simulink model "PhaseII_opalrt_NoProtection"  (Simulink 8.8)
settings: Solver=ode3  StartTime=0.0  StopTime=inf  FixedStep=Ts  RelTol=1e-5  EnableMultiTasking=on
PostLoadFcn:
  | %BESS ctrl
  | Kpf=0.005*3*12;
  | Kif=5*6;
  | 
  | Kpf1=0.005*3*12;
  | Kif1=5*6;
  | Kp_v=0.016*15*35;
  | Ki_v=12*25;
  | 
  | Kp_v1=0.016*15*35;
  | Ki_v1=12*25;
  | 
  | Vabc_B=12.47e3;
  | Vdc_ref=Vabc_B*2;
  | Kpwm=sqrt(2)*Vabc_B/Vdc_ref;
  | ZB=Vabc_B^2/1e6;
  | R=0.005*ZB;
  | Ibasefull=673/2*sqrt(2);
  | 
  | 
  | Ts_Control=1e-4;
  | ts=0.05;
  | delay=0.2;
  | offset=10e3;
  | t_plan=60;
  | t_monitor=.2;
  | t_mon=t_monitor;
  | scalingfactor=1;
  | x=0.5;
  | n=6;
  | %t_plan=1/15;
  | %t_monitor=10/900;
  | %t_mon=10/900;
  | 
  | %t_plan=1/5;
  | %t_monitor=10/300;
  | %t_mon=10/300;
  | %scalingfactor=1/300;
  | 
  | f0=60;
  | 
  | Pabc_B=1e6;
  | Iabc_B=Pabc_B*sqrt(2/3)/Vabc_B;  % pk value
  | Imax_1=2.5;
  | Ptrans_B=Pabc_B*200;
  | 
  | Vdc_ref=Vabc_B*2;
  | 
  | ZB=Vabc_B^2/Pabc_B;
  | L=0.1*ZB/2/pi/60;
  | R=0.1*ZB;
  | C=1/(4*pi^2*(2e3)^2*L);
  | 
  | LL=0.005*ZB/2/pi/60;
  | RR=0.005*ZB;
  | 
  | RC=0.02;
  | 
  | %%% Initial SOC %%%%
  | SOC_ini_BESS1=0.5;
  | ... (+223 lines)
InitFcn:
  | %BESS ctrl
  | Kpf=0.005*3*12;
  | Kif=5*6;
  | 
  | Kpf1=0.005*3*12;
  | Kif1=5*6;
  | Kp_v=0.016*15*35;
  | Ki_v=12*25;
  | 
  | Kp_v1=0.016*15*35;
  | Ki_v1=12*25;
  | 
  | Vabc_B=12.47e3;
  | Vdc_ref=Vabc_B*2;
  | Kpwm=sqrt(2)*Vabc_B/Vdc_ref;
  | ZB=Vabc_B^2/1e6;
  | R=0.005*ZB;
  | Ibasefull=673/2*sqrt(2);
  | 
  | 
  | Ts_Control=1e-4;
  | ts=0.05;
  | delay=0.2;
  | offset=10e3;
  | t_plan=60;
  | t_monitor=.2;
  | t_mon=t_monitor;
  | scalingfactor=1;
  | x=0.5;
  | n=6;
  | %t_plan=1/15;
  | %t_monitor=10/900;
  | %t_mon=10/900;
  | 
  | %t_plan=1/5;
  | %t_monitor=10/300;
  | %t_mon=10/300;
  | %scalingfactor=1/300;
  | 
  | f0=60;
  | 
  | Pabc_B=1e6;
  | Iabc_B=Pabc_B*sqrt(2/3)/Vabc_B;  % pk value
  | Imax_1=2.5;
  | Ptrans_B=Pabc_B*200;
  | 
  | Vdc_ref=Vabc_B*2;
  | 
  | ZB=Vabc_B^2/Pabc_B;
  | L=0.1*ZB/2/pi/60;
  | R=0.1*ZB;
  | C=1/(4*pi^2*(2e3)^2*L);
  | 
  | LL=0.005*ZB/2/pi/60;
  | RR=0.005*ZB;
  | 
  | RC=0.02;
  | 
  | %%% Initial SOC %%%%
  | SOC_ini_BESS1=0.5;
  | ... (+223 lines)
undefined symbols (not defined in the file): D1, Delta, DiscIntNeverNeededParam, Left, PG2ref, type, V
libraries: powerlib x220, powerlib_meascontrol x82, dspstat3 x54, dsparch4 x43, dspswit3 x24, simulink x19, simulink_extras x12, powerlib_extras x11, ssn_lib x7, artemis x6, rtlab x5, rtio_generic_dnp3 x5
(part 7 of 9)

== system PhaseII_opalrt_NoProtection/SM_System/Subsystem3/Fault ==
  In7 : Inport
  Breaker : powerlib/Elements/Breaker  InitialState=0  SwitchingTimes="[1/60  5/60]"  External=on  BreakerResistance=0.001  SnubberResistance=1e6  SnubberCapacitance=inf  Measurements=None  MoreParameters=on  NoBreakLoop=off
  Breaker1 : powerlib/Elements/Breaker  InitialState=0  SwitchingTimes="[1/60  5/60]"  External=on  BreakerResistance=0.001  SnubberResistance=1e6  SnubberCapacitance=inf  Measurements=None  MoreParameters=on  NoBreakLoop=off
  Breaker2 : powerlib/Elements/Breaker  InitialState=0  SwitchingTimes="[1/60  5/60]"  External=on  BreakerResistance=0.001  SnubberResistance=1e6  SnubberCapacitance=inf  Measurements=None  MoreParameters=on  NoBreakLoop=off
  In1 : PMIOPort  Port=1  Side=Left
  In2 : PMIOPort  Port=2  Side=Right
  In3 : PMIOPort  Port=3  Side=Left
  In4 : PMIOPort  Port=4  Side=Right
  In5 : PMIOPort  Port=5  Side=Left
  In6 : PMIOPort  Port=6  Side=Right
  wires:
  In7/1 -> Breaker1/1, Breaker2/1, Breaker/1
  connections:
  Breaker2/LConn1 -- In5/RConn1
  Breaker2/RConn1 -- In6/RConn1
  Breaker1/RConn1 -- In4/RConn1
  Breaker1/LConn1 -- In3/RConn1
  Breaker/RConn1 -- In2/RConn1
  Breaker/LConn1 -- In1/RConn1

== system PhaseII_opalrt_NoProtection/SM_System/Subsystem4/Fault ==
  In7 : Inport
  Breaker : powerlib/Elements/Breaker  InitialState=0  SwitchingTimes="[1/60  5/60]"  External=on  BreakerResistance=0.001  SnubberResistance=1e6  SnubberCapacitance=inf  Measurements=None  MoreParameters=on  NoBreakLoop=off
  Breaker1 : powerlib/Elements/Breaker  InitialState=0  SwitchingTimes="[1/60  5/60]"  External=on  BreakerResistance=0.001  SnubberResistance=1e6  SnubberCapacitance=inf  Measurements=None  MoreParameters=on  NoBreakLoop=off
  Breaker2 : powerlib/Elements/Breaker  InitialState=0  SwitchingTimes="[1/60  5/60]"  External=on  BreakerResistance=0.001  SnubberResistance=1e6  SnubberCapacitance=inf  Measurements=None  MoreParameters=on  NoBreakLoop=off
  In1 : PMIOPort  Port=1  Side=Left
  In2 : PMIOPort  Port=2  Side=Right
  In3 : PMIOPort  Port=3  Side=Left
  In4 : PMIOPort  Port=4  Side=Right
  In5 : PMIOPort  Port=5  Side=Left
  In6 : PMIOPort  Port=6  Side=Right
  wires:
  In7/1 -> Breaker/1, Breaker2/1, Breaker1/1
  connections:
  Breaker/LConn1 -- In1/RConn1
  Breaker/RConn1 -- In2/RConn1
  Breaker1/LConn1 -- In3/RConn1
  Breaker1/RConn1 -- In4/RConn1
  Breaker2/RConn1 -- In6/RConn1
  Breaker2/LConn1 -- In5/RConn1

== system PhaseII_opalrt_NoProtection/SS_LocalControl/BESS1/PI_Vd1 ==
  Error : Inport
  T_islanding : Inport  Port=2
  Add : Sum
  Add1 : Sum  Inputs=+-
  Constant25 : Constant  Value=4
  D2 : Scope  NumInputPorts=2
  Delay : Delay  DelayLength=1
  Embedded MATLAB Function1 : MATLAB Function  TreatAsAtomicUnit=on
  Integrator : Integrator  ExternalReset=rising  InitialConditionSource=external  LimitOutput=on  UpperSaturationLimit=Iabc_B*BESS_limit  LowerSaturationLimit=-Iabc_B*BESS_limit
  K : Gain
  K1 : Gain
  K2 : Gain  Gain=Vabc_B
  K3 : Gain  Gain=-1
  Ki1 : Gain  Gain=Kif/1.2
  Kp1 : Gain  Gain=Kpf/1.2
  Logical Operator : Logic  AllPortsSameDT=off  OutDataTypeStr=boolean
  PLL : powerlib_meascontrol/PLL/PLL  Fmin=58  Par_Init=[0, 60]  ParK=[180, 3200, 1]  TcD=1e-4  MaxRateChangeFreq=12  FilterCutOffFreq=25  Ts=0  AGC=on
  Relational Operator : RelationalOperator  Operator=<  OutDataTypeStr=boolean  ZeroCross=off  RndMeth=Nearest
  Relational Operator1 : RelationalOperator  Operator=>  OutDataTypeStr=boolean  ZeroCross=off  RndMeth=Nearest
  Out : Outport
  wires:
  K1/1 -> Relational Operator1/1, Relational Operator/1, Out/1
  Logical Operator/1 -> D2/1, Embedded MATLAB Function1/2(enable)
  Relational Operator/1 -> Logical Operator/1
  Relational Operator1/1 -> Logical Operator/2
  K3/1 -> Relational Operator1/2
  Embedded MATLAB Function1/1(dout) -> Integrator/1
  Add/1 -> K1/1
  K/1 -> Kp1/1, Ki1/1
  Ki1/1 -> Embedded MATLAB Function1/1(din)
  Kp1/1 -> Add1/2, Add/1
  Integrator/1 -> Add/2
  Constant25/1 -> K3/1, Relational Operator/2
  Error/1 -> D2/2, K/1
  T_islanding/1 -> Integrator/2
  Delay/1 -> Integrator/3
  [Ddg] -> Add1/1
  Add1/1 -> Delay/1

== system PhaseII_opalrt_NoProtection/SS_LocalControl/BESS1/PI_Vd10 ==
  Error : Inport
  T_islanding : Inport  Port=2
  Add : Sum
  Add1 : Sum  Inputs=+-
  Constant25 : Constant  Value=6
  D2 : Scope  NumInputPorts=2
  Delay : Delay  DelayLength=1
  Embedded MATLAB Function1 : MATLAB Function  TreatAsAtomicUnit=on
  Integrator1 : Integrator  ExternalReset=rising  InitialConditionSource=external  LimitOutput=on  UpperSaturationLimit=1  LowerSaturationLimit=-1
  K : Gain
  K1 : Gain
  K2 : Gain  Gain=Vabc_B
  K3 : Gain  Gain=-1
  Ki1 : Gain  Gain=Ki_v
  Kp1 : Gain  Gain=Kp_v
  Logical Operator : Logic  AllPortsSameDT=off  OutDataTypeStr=boolean
  PLL : powerlib_meascontrol/PLL/PLL  Fmin=58  Par_Init=[0, 60]  ParK=[180, 3200, 1]  TcD=1e-4  MaxRateChangeFreq=12  FilterCutOffFreq=25  Ts=0  AGC=on
  Relational Operator : RelationalOperator  Operator=<  OutDataTypeStr=boolean  ZeroCross=off  RndMeth=Nearest
  Relational Operator1 : RelationalOperator  Operator=>  OutDataTypeStr=boolean  ZeroCross=off  RndMeth=Nearest
  Out : Outport
  wires:
  Error/1 -> K/1, D2/2
  Constant25/1 -> Relational Operator/2, K3/1
  Integrator1/1 -> D2/1, Add/2
  Kp1/1 -> Add1/2, Add/1
  Ki1/1 -> Embedded MATLAB Function1/1(din)
  K/1 -> Ki1/1, Kp1/1
  Add/1 -> K1/1
  K3/1 -> Relational Operator1/2
  Relational Operator1/1 -> Logical Operator/2
  Relational Operator/1 -> Logical Operator/1
  Logical Operator/1 -> Embedded MATLAB Function1/2(enable)
  K1/1 -> Out/1, Relational Operator/1, Relational Operator1/1
  Embedded MATLAB Function1/1(dout) -> Integrator1/1
  T_islanding/1 -> Integrator1/2
  [Iq_ref_ini] -> Add1/1
  Add1/1 -> Delay/1
  Delay/1 -> Integrator1/3

== system PhaseII_opalrt_NoProtection/SS_LocalControl/BESS1/PI_Vd11 ==
  Error : Inport
  T_islanding : Inport  Port=2
  Add : Sum
  Add1 : Sum  Inputs=+-
  Constant25 : Constant  Value=4
  D2 : Scope  NumInputPorts=2
  Delay : Delay  DelayLength=1
  Embedded MATLAB Function1 : MATLAB Function  TreatAsAtomicUnit=on
  Integrator : Integrator  ExternalReset=rising  InitialConditionSource=external  LimitOutput=on  UpperSaturationLimit=Iabc_B*BESS_limit  LowerSaturationLimit=-Iabc_B*BESS_limit
  K : Gain
  K1 : Gain
  K2 : Gain  Gain=Vabc_B
  K3 : Gain  Gain=-1
  Ki1 : Gain  Gain=Kif/1.2
  Kp1 : Gain  Gain=Kpf/1.2
  Logical Operator : Logic  AllPortsSameDT=off  OutDataTypeStr=boolean
  PLL : powerlib_meascontrol/PLL/PLL  Fmin=58  Par_Init=[0, 60]  ParK=[180, 3200, 1]  TcD=1e-4  MaxRateChangeFreq=12  FilterCutOffFreq=25  Ts=0  AGC=on
  Relational Operator : RelationalOperator  Operator=<  OutDataTypeStr=boolean  ZeroCross=off  RndMeth=Nearest
  Relational Operator1 : RelationalOperator  Operator=>  OutDataTypeStr=boolean  ZeroCross=off  RndMeth=Nearest
  Out : Outport
  wires:
  K1/1 -> Relational Operator1/1, Relational Operator/1, Out/1
  Logical Operator/1 -> D2/1, Embedded MATLAB Function1/2(enable)
  Relational Operator/1 -> Logical Operator/1
  Relational Operator1/1 -> Logical Operator/2
  K3/1 -> Relational Operator1/2
  Embedded MATLAB Function1/1(dout) -> Integrator/1
  Add/1 -> K1/1
  K/1 -> Kp1/1, Ki1/1
  Ki1/1 -> Embedded MATLAB Function1/1(din)
  Kp1/1 -> Add1/2, Add/1
  Integrator/1 -> Add/2
  Constant25/1 -> K3/1, Relational Operator/2
  Error/1 -> D2/2, K/1
  T_islanding/1 -> Integrator/2
  Delay/1 -> Integrator/3
  [Dqg] -> Add1/1
  Add1/1 -> Delay/1

== system PhaseII_opalrt_NoProtection/SS_LocalControl/BESS1/PI_Vd2 ==
  Error : Inport
  Add : Sum
  Constant25 : Constant
  D2 : Scope  NumInputPorts=2
  Embedded MATLAB Function1 : MATLAB Function  TreatAsAtomicUnit=on
  Integrator : Integrator  ZeroCross=off
  K : Gain
  K1 : Gain
  K2 : Gain  Gain=Vabc_B
  K3 : Gain  Gain=-1
  Ki1 : Gain  Gain=Kif/1.2/1000
  Kp1 : Gain  Gain=Kpf/1.2
  Logical Operator : Logic  AllPortsSameDT=off  OutDataTypeStr=boolean
  PLL : powerlib_meascontrol/PLL/PLL  Fmin=58  Par_Init=[0, 60]  ParK=[180, 3200, 1]  TcD=1e-4  MaxRateChangeFreq=12  FilterCutOffFreq=25  Ts=0  AGC=on
  Relational Operator : RelationalOperator  Operator=<  OutDataTypeStr=boolean  ZeroCross=off  RndMeth=Nearest
  Relational Operator1 : RelationalOperator  Operator=>  OutDataTypeStr=boolean  ZeroCross=off  RndMeth=Nearest
  Out : Outport
  wires:
  K1/1 -> Relational Operator1/1, Relational Operator/1, Out/1
  Logical Operator/1 -> D2/1, Embedded MATLAB Function1/2(enable)
  Relational Operator/1 -> Logical Operator/1
  Relational Operator1/1 -> Logical Operator/2
  K3/1 -> Relational Operator1/2
  Embedded MATLAB Function1/1(dout) -> Integrator/1
  Add/1 -> K1/1
  K/1 -> Kp1/1, Ki1/1
  Ki1/1 -> Embedded MATLAB Function1/1(din)
  Kp1/1 -> Add/1
  Integrator/1 -> Add/2
  Constant25/1 -> K3/1, Relational Operator/2
  Error/1 -> D2/2, K/1

== system PhaseII_opalrt_NoProtection/SS_LocalControl/BESS1/PI_Vd3 ==
  Error : Inport
  Add : Sum
  Constant25 : Constant
  D2 : Scope  NumInputPorts=2
  Embedded MATLAB Function1 : MATLAB Function  TreatAsAtomicUnit=on
  Integrator : Integrator  ZeroCross=off
  K : Gain
  K1 : Gain
  K2 : Gain  Gain=Vabc_B
  K3 : Gain  Gain=-1
  Ki1 : Gain  Gain=Kif/1.2/1000
  Kp1 : Gain  Gain=Kpf/1.2
  Logical Operator : Logic  AllPortsSameDT=off  OutDataTypeStr=boolean
  PLL : powerlib_meascontrol/PLL/PLL  Fmin=58  Par_Init=[0, 60]  ParK=[180, 3200, 1]  TcD=1e-4  MaxRateChangeFreq=12  FilterCutOffFreq=25  Ts=0  AGC=on
  Relational Operator : RelationalOperator  Operator=<  OutDataTypeStr=boolean  ZeroCross=off  RndMeth=Nearest
  Relational Operator1 : RelationalOperator  Operator=>  OutDataTypeStr=boolean  ZeroCross=off  RndMeth=Nearest
  Out : Outport
  wires:
  K1/1 -> Relational Operator1/1, Relational Operator/1, Out/1
  Logical Operator/1 -> D2/1, Embedded MATLAB Function1/2(enable)
  Relational Operator/1 -> Logical Operator/1
  Relational Operator1/1 -> Logical Operator/2
  K3/1 -> Relational Operator1/2
  Embedded MATLAB Function1/1(dout) -> Integrator/1
  Add/1 -> K1/1
  K/1 -> Kp1/1, Ki1/1
  Ki1/1 -> Embedded MATLAB Function1/1(din)
  Kp1/1 -> Add/1
  Integrator/1 -> Add/2
  Constant25/1 -> K3/1, Relational Operator/2
  Error/1 -> D2/2, K/1

== system PhaseII_opalrt_NoProtection/SS_LocalControl/BESS1/PI_Vd5 ==
  Error : Inport
  Add : Sum
  Constant25 : Constant  Value=2
  D2 : Scope  NumInputPorts=2
  Embedded MATLAB Function1 : MATLAB Function  TreatAsAtomicUnit=on
  Integrator : Integrator  ZeroCross=off
  K : Gain
  K1 : Gain
  K2 : Gain  Gain=Vabc_B
  K3 : Gain  Gain=-1
  Ki1 : Gain  Gain=Ki_v
  Kp1 : Gain  Gain=Kp_v
  Logical Operator : Logic  AllPortsSameDT=off  OutDataTypeStr=boolean
  PLL : powerlib_meascontrol/PLL/PLL  Fmin=58  Par_Init=[0, 60]  ParK=[180, 3200, 1]  TcD=1e-4  MaxRateChangeFreq=12  FilterCutOffFreq=25  Ts=0  AGC=on
  Relational Operator : RelationalOperator  Operator=<  OutDataTypeStr=boolean  ZeroCross=off  RndMeth=Nearest
  Relational Operator1 : RelationalOperator  Operator=>  OutDataTypeStr=boolean  ZeroCross=off  RndMeth=Nearest
  Out : Outport
  wires:
  Error/1 -> K/1, D2/2
  Constant25/1 -> Relational Operator/2, K3/1
  Integrator/1 -> Add/2
  Kp1/1 -> Add/1
  Ki1/1 -> Embedded MATLAB Function1/1(din)
  K/1 -> Ki1/1, Kp1/1
  Add/1 -> K1/1
  Embedded MATLAB Function1/1(dout) -> Integrator/1
  K3/1 -> Relational Operator1/2
  Relational Operator1/1 -> Logical Operator/2
  Relational Operator/1 -> Logical Operator/1
  Logical Operator/1 -> Embedded MATLAB Function1/2(enable), D2/1
  K1/1 -> Out/1, Relational Operator/1, Relational Operator1/1

== system PhaseII_opalrt_NoProtection/SS_LocalControl/BESS1/PI_Vd6 ==
  Error : Inport
  Add : Sum
  Constant25 : Constant  Value=2
  D2 : Scope  NumInputPorts=2
  Embedded MATLAB Function1 : MATLAB Function  TreatAsAtomicUnit=on
  Integrator : Integrator  ZeroCross=off
  K : Gain
  K1 : Gain
  K2 : Gain  Gain=Vabc_B
  K3 : Gain  Gain=-1
  Ki1 : Gain  Gain=Ki_v
  Kp1 : Gain  Gain=Kp_v
  Logical Operator : Logic  AllPortsSameDT=off  OutDataTypeStr=boolean
  PLL : powerlib_meascontrol/PLL/PLL  Fmin=58  Par_Init=[0, 60]  ParK=[180, 3200, 1]  TcD=1e-4  MaxRateChangeFreq=12  FilterCutOffFreq=25  Ts=0  AGC=on
  Relational Operator : RelationalOperator  Operator=<  OutDataTypeStr=boolean  ZeroCross=off  RndMeth=Nearest
  Relational Operator1 : RelationalOperator  Operator=>  OutDataTypeStr=boolean  ZeroCross=off  RndMeth=Nearest
  Out : Outport
  wires:
  Error/1 -> K/1, D2/2
  Constant25/1 -> Relational Operator/2, K3/1
  Integrator/1 -> Add/2
  Kp1/1 -> Add/1
  Ki1/1 -> Embedded MATLAB Function1/1(din)
  K/1 -> Ki1/1, Kp1/1
  Add/1 -> K1/1
  Embedded MATLAB Function1/1(dout) -> Integrator/1
  K3/1 -> Relational Operator1/2
  Relational Operator1/1 -> Logical Operator/2
  Relational Operator/1 -> Logical Operator/1
  Logical Operator/1 -> Embedded MATLAB Function1/2(enable), D2/1
  K1/1 -> Out/1, Relational Operator/1, Relational Operator1/1

== system PhaseII_opalrt_NoProtection/SS_LocalControl/BESS1/PI_Vd7 ==
  Error : Inport
  T_islanding : Inport  Port=2
  Add : Sum
  Add1 : Sum  Inputs=+-
  Constant25 : Constant
  D2 : Scope  NumInputPorts=2
  Delay : Delay  DelayLength=1
  Embedded MATLAB Function1 : MATLAB Function  TreatAsAtomicUnit=on
  Integrator : Integrator  ExternalReset=falling  InitialConditionSource=external  LimitOutput=on  UpperSaturationLimit=Iabc_B*BESS_limit  LowerSaturationLimit=-Iabc_B*BESS_limit
  K : Gain
  K1 : Gain
  K2 : Gain  Gain=Vabc_B
  K3 : Gain  Gain=-1
  Ki1 : Gain  Gain=Kif
  Kp1 : Gain  Gain=Kpf
  Logical Operator : Logic  AllPortsSameDT=off  OutDataTypeStr=boolean
  PLL : powerlib_meascontrol/PLL/PLL  Fmin=58  Par_Init=[0, 60]  ParK=[180, 3200, 1]  TcD=1e-4  MaxRateChangeFreq=12  FilterCutOffFreq=25  Ts=0  AGC=on
  Relational Operator : RelationalOperator  Operator=<  OutDataTypeStr=boolean  ZeroCross=off  RndMeth=Nearest
  Relational Operator1 : RelationalOperator  Operator=>  OutDataTypeStr=boolean  ZeroCross=off  RndMeth=Nearest
  Out : Outport
  wires:
  K1/1 -> Relational Operator1/1, Relational Operator/1, Out/1
  Logical Operator/1 -> D2/1, Embedded MATLAB Function1/2(enable)
  Relational Operator/1 -> Logical Operator/1
  Relational Operator1/1 -> Logical Operator/2
  K3/1 -> Relational Operator1/2
  Embedded MATLAB Function1/1(dout) -> Integrator/1
  Add/1 -> K1/1
  K/1 -> Kp1/1, Ki1/1
  Ki1/1 -> Embedded MATLAB Function1/1(din)
  Kp1/1 -> Add1/2, Add/1
  Integrator/1 -> Add/2
  Constant25/1 -> K3/1, Relational Operator/2
  Error/1 -> D2/2, K/1
  T_islanding/1 -> Integrator/2
  Delay/1 -> Integrator/3
  [Ddi] -> Add1/1
  Add1/1 -> Delay/1

== system PhaseII_opalrt_NoProtection/SS_LocalControl/BESS1/PI_Vd8 ==
  Error : Inport
  T_islanding : Inport  Port=2
  Add : Sum
  Add1 : Sum  Inputs=+-
  Constant25 : Constant  Value=4
  D2 : Scope  NumInputPorts=2
  Delay : Delay  DelayLength=1
  Embedded MATLAB Function1 : MATLAB Function  TreatAsAtomicUnit=on
  Integrator1 : Integrator  ExternalReset=rising  InitialConditionSource=external  LimitOutput=on  UpperSaturationLimit=2.2  LowerSaturationLimit=-2.2
  K : Gain
  K1 : Gain
  K2 : Gain  Gain=Vabc_B
  K3 : Gain  Gain=-1
  Ki1 : Gain  Gain=Ki_v
  Kp1 : Gain  Gain=Kp_v
  Logical Operator : Logic  AllPortsSameDT=off  OutDataTypeStr=boolean
  PLL : powerlib_meascontrol/PLL/PLL  Fmin=58  Par_Init=[0, 60]  ParK=[180, 3200, 1]  TcD=1e-4  MaxRateChangeFreq=12  FilterCutOffFreq=25  Ts=0  AGC=on
  Relational Operator : RelationalOperator  Operator=<  OutDataTypeStr=boolean  ZeroCross=off  RndMeth=Nearest
  Relational Operator1 : RelationalOperator  Operator=>  OutDataTypeStr=boolean  ZeroCross=off  RndMeth=Nearest
  Out : Outport
  wires:
  Error/1 -> K/1, D2/2
  Constant25/1 -> Relational Operator/2, K3/1
  Integrator1/1 -> D2/1, Add/2
  Kp1/1 -> Add1/2, Add/1
  Ki1/1 -> Embedded MATLAB Function1/1(din)
  K/1 -> Ki1/1, Kp1/1
  Add/1 -> K1/1
  K3/1 -> Relational Operator1/2
  Relational Operator1/1 -> Logical Operator/2
  Relational Operator/1 -> Logical Operator/1
  Logical Operator/1 -> Embedded MATLAB Function1/2(enable)
  K1/1 -> Out/1, Relational Operator/1, Relational Operator1/1
  Embedded MATLAB Function1/1(dout) -> Integrator1/1
  T_islanding/1 -> Integrator1/2
  [Id_ref_ini] -> Add1/1
  Add1/1 -> Delay/1
  Delay/1 -> Integrator1/3

== system PhaseII_opalrt_NoProtection/SS_LocalControl/BESS1/PI_Vd9 ==
  Error : Inport
  T_islanding : Inport  Port=2
  Add : Sum
  Add1 : Sum  Inputs=+-
  Constant25 : Constant
  D2 : Scope  NumInputPorts=2
  Delay : Delay  DelayLength=1
  Embedded MATLAB Function1 : MATLAB Function  TreatAsAtomicUnit=on
  Integrator : Integrator  ExternalReset=falling  InitialConditionSource=external  LimitOutput=on  UpperSaturationLimit=Iabc_B*BESS_limit  LowerSaturationLimit=-Iabc_B*BESS_limit
  K : Gain
  K1 : Gain
  K2 : Gain  Gain=Vabc_B
  K3 : Gain  Gain=-1
  Ki1 : Gain  Gain=Kif
  Kp1 : Gain  Gain=Kpf
  Logical Operator : Logic  AllPortsSameDT=off  OutDataTypeStr=boolean
  PLL : powerlib_meascontrol/PLL/PLL  Fmin=58  Par_Init=[0, 60]  ParK=[180, 3200, 1]  TcD=1e-4  MaxRateChangeFreq=12  FilterCutOffFreq=25  Ts=0  AGC=on
  Relational Operator : RelationalOperator  Operator=<  OutDataTypeStr=boolean  ZeroCross=off  RndMeth=Nearest
  Relational Operator1 : RelationalOperator  Operator=>  OutDataTypeStr=boolean  ZeroCross=off  RndMeth=Nearest
  Out : Outport
  wires:
  K1/1 -> Relational Operator1/1, Relational Operator/1, Out/1
  Logical Operator/1 -> D2/1, Embedded MATLAB Function1/2(enable)
  Relational Operator/1 -> Logical Operator/1
  Relational Operator1/1 -> Logical Operator/2
  K3/1 -> Relational Operator1/2
  Embedded MATLAB Function1/1(dout) -> Integrator/1
  Add/1 -> K1/1
  K/1 -> Kp1/1, Ki1/1
  Ki1/1 -> Embedded MATLAB Function1/1(din)
  Kp1/1 -> Add1/2, Add/1
  Integrator/1 -> Add/2
  Constant25/1 -> K3/1, Relational Operator/2
  Error/1 -> D2/2, K/1
  T_islanding/1 -> Integrator/2
  Delay/1 -> Integrator/3
  [Dqi] -> Add1/1
  Add1/1 -> Delay/1

== system PhaseII_opalrt_NoProtection/SS_LocalControl/BESS1/SW Command ==
  f : Inport
  Vd : Inport  Port=2
  SW_Ctr : Inport  Port=3
  Abs2 : Abs
  Abs3 : Abs
  Add3 : Sum  Inputs=+-
  Add4 : Sum  Inputs=+-
  Constant1 : Constant  Value=5
  Constant2 : Constant
  Constant20 : Constant  Value=0.15
  Constant21 : Constant  Value=.2
  Constant22 : Constant
  Constant23 : Constant  Value=60
  Conv : DataTypeConversion  OutDataTypeStr=double
  Counter : dspswit3/Counter  Direction=Up  CountEvent=Non-zero sample  CounterSize=User defined  MaxCount=255  InitialCount=0  Output=Hit  HitValue=50  ResetInput=on  SamplesPerFrame=1  Ts=1  CntDtype=double  HitDtype=Logical
  Counter1 : dspswit3/Counter  Direction=Up  CountEvent=Rising edge  CounterSize=User defined  MaxCount=255  InitialCount=0  Output=Count  HitValue=50  ResetInput=on  SamplesPerFrame=1  Ts=1  CntDtype=double  HitDtype=Logical
  D Latch2 : simulink_extras/Flip Flops/D Latch
  D1 : Scope  NumInputPorts=3
  D8 : Scope  NumInputPorts=3
  Delay : Delay  DelayLength=1
  Logical Operator : Logic  AllPortsSameDT=off  OutDataTypeStr=boolean
  Logical Operator{1..3,5} (4 alike) : Logic  Operator=NOT  AllPortsSameDT=off  OutDataTypeStr=boolean
  Logical Operator4 : Logic  Operator=OR  AllPortsSameDT=off  OutDataTypeStr=boolean
  Memory : Memory
  Relational Operator1 : RelationalOperator  OutDataTypeStr=boolean  RndMeth=Nearest
  Relational Operator2 : RelationalOperator  OutDataTypeStr=boolean  RndMeth=Nearest
  Relational Operator3 : RelationalOperator  OutDataTypeStr=boolean  RndMeth=Nearest
  SW_Cmd : Outport
  wires:
  Abs2/1 -> Relational Operator2/1
  Add3/1 -> Abs2/1
  Constant23/1 -> Add3/2
  Constant21/1 -> Relational Operator2/2
  Relational Operator2/1 -> D1/1, Logical Operator4/1
  Add4/1 -> Abs3/1
  Constant22/1 -> Add4/2
  D Latch2/1 -> D8/3, Logical Operator2/1
  Relational Operator3/1 -> D1/2, Logical Operator4/2
  Abs3/1 -> Relational Operator3/1
  Constant20/1 -> Relational Operator3/2
  Constant1/1 -> Relational Operator1/2
  Counter/1 -> Counter1/1
  Counter1/1 -> D1/3, Relational Operator1/1
  Logical Operator1/1 -> Counter/2
  Logical Operator4/1 -> Logical Operator5/1, Logical Operator1/1, Counter/1
  Conv/1 -> Memory/1
  SW_Ctr/1 -> Delay/1
  Logical Operator/1 -> Conv/1
  Logical Operator2/1 -> Logical Operator/1
  Relational Operator1/1 -> D Latch2/1
  Delay/1 -> D8/2, Logical Operator/2
  Logical Operator5/1 -> Counter1/2
  Constant2/1 -> D Latch2/2
  Vd/1 -> Add4/1
  f/1 -> Add3/1
  Memory/1 -> Logical Operator3/1, D8/1
  Logical Operator3/1 -> SW_Cmd/1

== system PhaseII_opalrt_NoProtection/SS_LocalControl/BESS1/Sequence decomposition ==
  abc : Inport
  Phase : Inport  Port=2
  Add : Sum  Inputs=+++
  Add1 : Sum
  Add2 : Sum  Inputs=+-
  Add3 : Sum
  Add4 : Sum  Inputs=-+
  Alpha-Beta-Zero to dq0 : powerlib_meascontrol/Transformations/Alpha-Beta-Zero to dq0  Alignment=90 degrees behind phase A axis
  Alpha-Beta-Zero to dq1 : powerlib_meascontrol/Transformations/Alpha-Beta-Zero to dq0  Alignment=90 degrees behind phase A axis
  Delay : Delay  DelayLength=42  InitialCondition=0
  Delay1 : Delay  DelayLength=42  InitialCondition=0
  Demux1 : Demux  Outputs=2
  Demux4 : Demux  Outputs=3
  Fcn3 : Fcn  Expr=sqrt(2/3)*(u[1]-u[2]*1/2-u[3]*1/2)
  Fcn5 : Fcn  Expr=sqrt(2/3)*(u[2]*sqrt(3)/2-u[3]*sqrt(3)/2)
  Gain1 : Gain  Gain=-1
  Gain2 : Gain  Gain=1/3
  Gain3 : Gain
  Gain{6..9} (4 alike) : Gain  Gain=1/2
  Mux : Mux  Inputs=3
  Mux1 : Mux  Inputs=3
  Mux2 : Mux  Inputs=2
  Mux3 : Mux  Inputs=3
  Pos_dq : Outport
  Neg_dq : Outport  Port=2
  zero : Outport  Port=3
  wires:
  Demux1/1 -> Add2/1, Add3/1, Delay/1
  Mux2/1 -> Demux1/1
  Demux1/2 -> Delay1/1, Add4/2, Add1/1
  Mux/1 -> Alpha-Beta-Zero to dq1/1
  Gain1/1 -> Alpha-Beta-Zero to dq1/2
  Alpha-Beta-Zero to dq0/1 -> Pos_dq/1
  Alpha-Beta-Zero to dq1/1 -> Neg_dq/1
  abc/1 -> Demux4/1
  Demux4/1 -> Mux1/1, Add/1
  Demux4/2 -> Mux1/2, Add/3
  Demux4/3 -> Mux1/3, Add/2
  Delay1/1 -> Add2/2, Add3/2
  Delay/1 -> Add4/1, Add1/2
  Add1/1 -> Gain7/1
  Add2/1 -> Gain6/1
  Add4/1 -> Gain9/1
  Add3/1 -> Gain8/1
  Gain8/1 -> Mux/1
  Gain9/1 -> Mux/2
  Mux3/1 -> Alpha-Beta-Zero to dq0/1
  Gain6/1 -> Mux3/1
  Gain7/1 -> Mux3/2
  Add/1 -> Gain2/1, Gain3/1
  Gain2/1 -> zero/1
  Phase/1 -> Gain1/1, Alpha-Beta-Zero to dq0/2
  Gain3/1 -> Mux3/3, Mux/3
  Mux1/1 -> Fcn3/1, Fcn5/1
  Fcn3/1 -> Mux2/1
  Fcn5/1 -> Mux2/2

== system PhaseII_opalrt_NoProtection/SS_LocalControl/BESS1/Sequence decomposition1 ==
  abc : Inport
  Phase : Inport  Port=2
  Add : Sum  Inputs=+++
  Add1 : Sum
  Add2 : Sum  Inputs=+-
  Add3 : Sum
  Add4 : Sum  Inputs=-+
  Alpha-Beta-Zero to dq0 : powerlib_meascontrol/Transformations/Alpha-Beta-Zero to dq0  Alignment=90 degrees behind phase A axis
  Alpha-Beta-Zero to dq1 : powerlib_meascontrol/Transformations/Alpha-Beta-Zero to dq0  Alignment=90 degrees behind phase A axis
  Delay : Delay  DelayLength=42  InitialCondition=0
  Delay1 : Delay  DelayLength=42  InitialCondition=0
  Demux1 : Demux  Outputs=2
  Demux4 : Demux  Outputs=3
  Fcn3 : Fcn  Expr=sqrt(2/3)*(u[1]-u[2]*1/2-u[3]*1/2)
  Fcn5 : Fcn  Expr=sqrt(2/3)*(u[2]*sqrt(3)/2-u[3]*sqrt(3)/2)
  Gain1 : Gain  Gain=-1
  Gain2 : Gain  Gain=1/3
  Gain3 : Gain
  Gain{6..9} (4 alike) : Gain  Gain=1/2
  Mux : Mux  Inputs=3
  Mux1 : Mux  Inputs=3
  Mux2 : Mux  Inputs=2
  Mux3 : Mux  Inputs=3
  Pos_dq : Outport
  Neg_dq : Outport  Port=2
  zero : Outport  Port=3
  wires:
  Fcn5/1 -> Mux2/2
  Fcn3/1 -> Mux2/1
  Mux1/1 -> Fcn5/1, Fcn3/1
  Gain3/1 -> Mux/3, Mux3/3
  Phase/1 -> Alpha-Beta-Zero to dq0/2, Gain1/1
  Gain2/1 -> zero/1
  Add/1 -> Gain3/1, Gain2/1
  Gain7/1 -> Mux3/2
  Gain6/1 -> Mux3/1
  Mux3/1 -> Alpha-Beta-Zero to dq0/1
  Gain9/1 -> Mux/2
  Gain8/1 -> Mux/1
  Add3/1 -> Gain8/1
  Add4/1 -> Gain9/1
  Add2/1 -> Gain6/1
  Add1/1 -> Gain7/1
  Delay/1 -> Add1/2, Add4/1
  Delay1/1 -> Add3/2, Add2/2
  Demux4/3 -> Add/2, Mux1/3
  Demux4/2 -> Add/3, Mux1/2
  Demux4/1 -> Add/1, Mux1/1
  abc/1 -> Demux4/1
  Alpha-Beta-Zero to dq1/1 -> Neg_dq/1
  Alpha-Beta-Zero to dq0/1 -> Pos_dq/1
  Gain1/1 -> Alpha-Beta-Zero to dq1/2
  Mux/1 -> Alpha-Beta-Zero to dq1/1
  Demux1/2 -> Add1/1, Add4/2, Delay1/1
  Mux2/1 -> Demux1/1
  Demux1/1 -> Delay/1, Add3/1, Add2/1

== system PhaseII_opalrt_NoProtection/SS_LocalControl/BESS1/Subsystem ==
  I_RMS : Inport
  Add : Sum  Inputs=+-
  Constant : Constant  Value=SOC_ini_BESS2*AH*3600
  Constant1 : Constant
  Gain : Gain  Gain=1/3600
  Gain3 : Gain  Gain=1/(AH*3600)
  Gain8 : Gain
  Integrator : Integrator
  Integrator1 : Integrator  InitialConditionSource=external  LimitOutput=on  UpperSaturationLimit=AH*3600  LowerSaturationLimit=0
  Battery_Ah : Outport
  Battery_SOC : Outport  Port=2
  wires:
  Gain8/1 -> Battery_SOC/1
  Gain/1 -> Battery_Ah/1
  I_RMS/1 -> Integrator1/1, Integrator/1
  Constant/1 -> Integrator1/2
  Add/1 -> Gain8/1
  Constant1/1 -> Add/1
  Gain3/1 -> Add/2
  Integrator1/1 -> Gain3/1
  Integrator/1 -> Gain/1

== system PhaseII_opalrt_NoProtection/SS_LocalControl/BESS1/V_theta_generation ==
  Pin : Inport
  Qin : Inport  Port=2
  Pin1 : Inport  Port=3
  "  " : Constant  Value=2*pi
  2 kHz1 : dsparch4/Analog Filter Design  method=Butterworth  filttype=Lowpass  N=2  Wlo=2*pi*0.1  Whi=80  Rp=2  Rs=40
  Constant1 : Constant  Value=1.64368  OutDataTypeStr=single
  D1 : Scope  Commented=on
  D{2..5,7} (5 alike) : Scope
  Delay : Delay  DelayLength=1  SampleTime=Ts
  Gain1 : Gain
  Gain2 : Gain  Gain=2*pi
  Gain3 : Gain
  Gain4 : Gain  Gain=1/2/pi
  Gain5 : Gain  Gain=1/2/pi
  Gain6 : Gain
  Gain7 : Gain  Gain=1/2/pi
  Gain8 : Gain  Gain=0
  Integrator : Integrator  ExternalReset=rising  InitialConditionSource=external  LimitOutput=on
  Kv : Constant  Value=0.1
  Math Function : Math  Operator=mod  SaturateOnIntegerOverflow=on
  P1 : Constant  Value=0.5
  P4 : Constant  Value=0
  P5 : Constant  Value=0.01
  Product : Product
  Product1 : Product
  Product2 : Product
  Q : Constant  Value=0
  Sum1 : Sum  Inputs=|-+
  Sum10 : Sum  Inputs=|++
  Sum13 : Sum  Inputs=+++
  Sum2 : Sum  Inputs=++++
  Sum3 : Sum  Inputs=|-+
  Sum4 : Sum
  V : Constant
  intergral : DiscreteTransferFcn  Commented=on  Numerator=Ts_Control/10  Denominator=[1 -1]  SampleTime=Ts_Control/10
  w0 : Constant  Value=60*2*pi
  w2 : Constant  Value=0
  Magd : Outport
  theta : Outport  Port=2
  Magq : Outport  Port=3
  frequency : Outport  Port=4
  tag scope: Phase_islanded_ref=global
  wires:
  Sum10/1 -> Product/2
  w0/1 -> Sum13/1
  Product/1 -> Gain2/1
  [Pba_ref] -> Sum10/1
  Sum13/1 -> Gain4/1, Integrator/1
  "  "/1 -> Math Function/2
  Math Function/1 -> D3/1, theta/1
  Gain3/1 -> Gain8/1, Sum10/2
  Pin/1 -> Gain3/1
  Integrator/1 -> [Phase_islanded_ref], D5/1, Math Function/1
  P1/1 -> Product/1
  Gain2/1 -> Sum13/2
  Gain1/1 -> Sum2/2
  Kv/1 -> Product1/1
  Sum1/1 -> Product1/2
  Sum2/1 -> D2/1, Magd/1, Gain5/1
  V/1 -> Sum2/1
  Q/1 -> Sum1/1
  Product1/1 -> Gain1/1
  Qin/1 -> Sum3/2, Sum1/2
  Gain6/1 -> Sum4/2
  Product2/1 -> Gain6/1
  P5/1 -> Product2/1
  Sum3/1 -> Product2/2
  Sum4/1 -> D4/1, Magq/1, Gain7/1
  P4/1 -> Sum3/1
  w2/1 -> Sum4/1
  Gain4/1 -> frequency/1, D7/1
  Pin1/1 -> Integrator/2
  [Phase_grid1] -> Delay/1
  Delay/1 -> Integrator/3
  [Fba_ref] -> Sum13/3
  [Vba_ref] -> Sum2/3
  Gain8/1 -> 2 kHz1/1
  2 kHz1/1 -> Sum2/4

== system PhaseII_opalrt_NoProtection/SS_LocalControl/BESS2/PI_Vd1 ==
  Error : Inport
  T_islanding : Inport  Port=2
  Add : Sum
  Add1 : Sum  Inputs=+-
  Constant25 : Constant  Value=4
  D2 : Scope  NumInputPorts=2
  Delay : Delay  DelayLength=1
  Embedded MATLAB Function1 : MATLAB Function  TreatAsAtomicUnit=on
  Integrator : Integrator  ExternalReset=rising  InitialConditionSource=external  LimitOutput=on  UpperSaturationLimit=Iabc_B*BESS_limit  LowerSaturationLimit=-Iabc_B*BESS_limit
  K : Gain
  K1 : Gain
  K2 : Gain  Gain=Vabc_B
  K3 : Gain  Gain=-1
  Ki1 : Gain  Gain=Kif/1.2
  Kp1 : Gain  Gain=Kpf/1.2
  Logical Operator : Logic  AllPortsSameDT=off  OutDataTypeStr=boolean
  PLL : powerlib_meascontrol/PLL/PLL  Fmin=58  Par_Init=[0, 60]  ParK=[180, 3200, 1]  TcD=1e-4  MaxRateChangeFreq=12  FilterCutOffFreq=25  Ts=0  AGC=on
  Relational Operator : RelationalOperator  Operator=<  OutDataTypeStr=boolean  ZeroCross=off  RndMeth=Nearest
  Relational Operator1 : RelationalOperator  Operator=>  OutDataTypeStr=boolean  ZeroCross=off  RndMeth=Nearest
  Out : Outport
  wires:
  K1/1 -> Relational Operator1/1, Relational Operator/1, Out/1
  Logical Operator/1 -> D2/1, Embedded MATLAB Function1/2(enable)
  Relational Operator/1 -> Logical Operator/1
  Relational Operator1/1 -> Logical Operator/2
  K3/1 -> Relational Operator1/2
  Embedded MATLAB Function1/1(dout) -> Integrator/1
  Add/1 -> K1/1
  K/1 -> Kp1/1, Ki1/1
  Ki1/1 -> Embedded MATLAB Function1/1(din)
  Kp1/1 -> Add1/2, Add/1
  Integrator/1 -> Add/2
  Constant25/1 -> K3/1, Relational Operator/2
  Error/1 -> D2/2, K/1
  Delay/1 -> Integrator/3
  [Ddg1] -> Add1/1
  Add1/1 -> Delay/1
  T_islanding/1 -> Integrator/2

== system PhaseII_opalrt_NoProtection/SS_LocalControl/BESS2/PI_Vd10 ==
  Error : Inport
  T_islanding : Inport  Port=2
  Add : Sum
  Add1 : Sum  Inputs=+-
  Constant25 : Constant  Value=2.2
  D2 : Scope  NumInputPorts=2
  Delay : Delay  DelayLength=1
  Embedded MATLAB Function1 : MATLAB Function  TreatAsAtomicUnit=on
  Integrator1 : Integrator  ExternalReset=rising  InitialConditionSource=external  LimitOutput=on  UpperSaturationLimit=2.2  LowerSaturationLimit=-2.2
  K : Gain
  K1 : Gain
  K2 : Gain  Gain=Vabc_B
  K3 : Gain  Gain=-1
  Ki1 : Gain  Gain=Ki_v
  Kp1 : Gain  Gain=Kp_v
  Logical Operator : Logic  AllPortsSameDT=off  OutDataTypeStr=boolean
  PLL : powerlib_meascontrol/PLL/PLL  Fmin=58  Par_Init=[0, 60]  ParK=[180, 3200, 1]  TcD=1e-4  MaxRateChangeFreq=12  FilterCutOffFreq=25  Ts=0  AGC=on
  Relational Operator : RelationalOperator  Operator=<  OutDataTypeStr=boolean  ZeroCross=off  RndMeth=Nearest
  Relational Operator1 : RelationalOperator  Operator=>  OutDataTypeStr=boolean  ZeroCross=off  RndMeth=Nearest
  Out : Outport
  wires:
  Error/1 -> K/1, D2/2
  Constant25/1 -> Relational Operator/2, K3/1
  Integrator1/1 -> D2/1, Add/2
  Kp1/1 -> Add1/2, Add/1
  Ki1/1 -> Embedded MATLAB Function1/1(din)
  K/1 -> Ki1/1, Kp1/1
  Add/1 -> K1/1
  K3/1 -> Relational Operator1/2
  Relational Operator1/1 -> Logical Operator/2
  Relational Operator/1 -> Logical Operator/1
  Logical Operator/1 -> Embedded MATLAB Function1/2(enable)
  K1/1 -> Out/1, Relational Operator/1, Relational Operator1/1
  Embedded MATLAB Function1/1(dout) -> Integrator1/1
  T_islanding/1 -> Integrator1/2
  [Id_ref_ini1] -> Add1/1
  Add1/1 -> Delay/1
  Delay/1 -> Integrator1/3

== system PhaseII_opalrt_NoProtection/SS_LocalControl/BESS2/PI_Vd2 ==
  Error : Inport
  Add : Sum
  Constant25 : Constant
  D2 : Scope  NumInputPorts=2
  Embedded MATLAB Function1 : MATLAB Function  TreatAsAtomicUnit=on
  Integrator : Integrator  ZeroCross=off
  K : Gain
  K1 : Gain
  K2 : Gain  Gain=Vabc_B
  K3 : Gain  Gain=-1
  Ki1 : Gain  Gain=Kif/1.2
  Kp1 : Gain  Gain=Kpf/1.2
  Logical Operator : Logic  AllPortsSameDT=off  OutDataTypeStr=boolean
  PLL : powerlib_meascontrol/PLL/PLL  Fmin=58  Par_Init=[0, 60]  ParK=[180, 3200, 1]  TcD=1e-4  MaxRateChangeFreq=12  FilterCutOffFreq=25  Ts=0  AGC=on
  Relational Operator : RelationalOperator  Operator=<  OutDataTypeStr=boolean  ZeroCross=off  RndMeth=Nearest
  Relational Operator1 : RelationalOperator  Operator=>  OutDataTypeStr=boolean  ZeroCross=off  RndMeth=Nearest
  Out : Outport
  wires:
  K1/1 -> Relational Operator1/1, Relational Operator/1, Out/1
  Logical Operator/1 -> D2/1, Embedded MATLAB Function1/2(enable)
  Relational Operator/1 -> Logical Operator/1
  Relational Operator1/1 -> Logical Operator/2
  K3/1 -> Relational Operator1/2
  Embedded MATLAB Function1/1(dout) -> Integrator/1
  Add/1 -> K1/1
  K/1 -> Kp1/1, Ki1/1
  Ki1/1 -> Embedded MATLAB Function1/1(din)
  Kp1/1 -> Add/1
  Integrator/1 -> Add/2
  Constant25/1 -> K3/1, Relational Operator/2
  Error/1 -> D2/2, K/1

== system PhaseII_opalrt_NoProtection/SS_LocalControl/BESS2/PI_Vd3 ==
  Error : Inport
  Add : Sum
  Constant25 : Constant
  D2 : Scope  NumInputPorts=2
  Embedded MATLAB Function1 : MATLAB Function  TreatAsAtomicUnit=on
  Integrator : Integrator  ZeroCross=off
  K : Gain
  K1 : Gain
  K2 : Gain  Gain=Vabc_B
  K3 : Gain  Gain=-1
  Ki1 : Gain  Gain=Kif/1.2
  Kp1 : Gain  Gain=Kpf/1.2
  Logical Operator : Logic  AllPortsSameDT=off  OutDataTypeStr=boolean
  PLL : powerlib_meascontrol/PLL/PLL  Fmin=58  Par_Init=[0, 60]  ParK=[180, 3200, 1]  TcD=1e-4  MaxRateChangeFreq=12  FilterCutOffFreq=25  Ts=0  AGC=on
  Relational Operator : RelationalOperator  Operator=<  OutDataTypeStr=boolean  ZeroCross=off  RndMeth=Nearest
  Relational Operator1 : RelationalOperator  Operator=>  OutDataTypeStr=boolean  ZeroCross=off  RndMeth=Nearest
  Out : Outport
  wires:
  K1/1 -> Relational Operator1/1, Relational Operator/1, Out/1
  Logical Operator/1 -> D2/1, Embedded MATLAB Function1/2(enable)
  Relational Operator/1 -> Logical Operator/1
  Relational Operator1/1 -> Logical Operator/2
  K3/1 -> Relational Operator1/2
  Embedded MATLAB Function1/1(dout) -> Integrator/1
  Add/1 -> K1/1
  K/1 -> Kp1/1, Ki1/1
  Ki1/1 -> Embedded MATLAB Function1/1(din)
  Kp1/1 -> Add/1
  Integrator/1 -> Add/2
  Constant25/1 -> K3/1, Relational Operator/2
  Error/1 -> D2/2, K/1

== system PhaseII_opalrt_NoProtection/SS_LocalControl/BESS2/PI_Vd4 ==
  Error : Inport
  T_islanding : Inport  Port=2
  Add : Sum
  Add1 : Sum  Inputs=+-
  Constant25 : Constant  Value=4
  D2 : Scope  NumInputPorts=2
  Delay : Delay  DelayLength=1
  Embedded MATLAB Function1 : MATLAB Function  TreatAsAtomicUnit=on
  Integrator : Integrator  ExternalReset=rising  InitialConditionSource=external  LimitOutput=on  UpperSaturationLimit=Iabc_B*BESS_limit  LowerSaturationLimit=-Iabc_B*BESS_limit
  K : Gain
  K1 : Gain
  K2 : Gain  Gain=Vabc_B
  K3 : Gain  Gain=-1
  Ki1 : Gain  Gain=Kif/1.2
  Kp1 : Gain  Gain=Kpf/1.2
  Logical Operator : Logic  AllPortsSameDT=off  OutDataTypeStr=boolean
  PLL : powerlib_meascontrol/PLL/PLL  Fmin=58  Par_Init=[0, 60]  ParK=[180, 3200, 1]  TcD=1e-4  MaxRateChangeFreq=12  FilterCutOffFreq=25  Ts=0  AGC=on
  Relational Operator : RelationalOperator  Operator=<  OutDataTypeStr=boolean  ZeroCross=off  RndMeth=Nearest
  Relational Operator1 : RelationalOperator  Operator=>  OutDataTypeStr=boolean  ZeroCross=off  RndMeth=Nearest
  Out : Outport
  wires:
  K1/1 -> Relational Operator1/1, Relational Operator/1, Out/1
  Logical Operator/1 -> D2/1, Embedded MATLAB Function1/2(enable)
  Relational Operator/1 -> Logical Operator/1
  Relational Operator1/1 -> Logical Operator/2
  K3/1 -> Relational Operator1/2
  Embedded MATLAB Function1/1(dout) -> Integrator/1
  Add/1 -> K1/1
  K/1 -> Kp1/1, Ki1/1
  Ki1/1 -> Embedded MATLAB Function1/1(din)
  Kp1/1 -> Add1/2, Add/1
  Integrator/1 -> Add/2
  Constant25/1 -> K3/1, Relational Operator/2
  Error/1 -> D2/2, K/1
  Delay/1 -> Integrator/3
  [Dqg1] -> Add1/1
  Add1/1 -> Delay/1
  T_islanding/1 -> Integrator/2

== system PhaseII_opalrt_NoProtection/SS_LocalControl/BESS2/PI_Vd5 ==
  Error : Inport
  Add : Sum
  Constant25 : Constant  Value=0.15
  D2 : Scope  NumInputPorts=2
  Embedded MATLAB Function1 : MATLAB Function  TreatAsAtomicUnit=on
  Integrator : Integrator  ZeroCross=off
  K : Gain
  K1 : Gain
  K2 : Gain  Gain=Vabc_B
  K3 : Gain  Gain=-1
  Ki1 : Gain  Gain=Ki_v
  Kp1 : Gain  Gain=Kp_v
  Logical Operator : Logic  AllPortsSameDT=off  OutDataTypeStr=boolean
  PLL : powerlib_meascontrol/PLL/PLL  Fmin=58  Par_Init=[0, 60]  ParK=[180, 3200, 1]  TcD=1e-4  MaxRateChangeFreq=12  FilterCutOffFreq=25  Ts=0  AGC=on
  Relational Operator : RelationalOperator  Operator=<  OutDataTypeStr=boolean  ZeroCross=off  RndMeth=Nearest
  Relational Operator1 : RelationalOperator  Operator=>  OutDataTypeStr=boolean  ZeroCross=off  RndMeth=Nearest
  Out : Outport
  wires:
  Error/1 -> K/1, D2/2
  Constant25/1 -> Relational Operator/2, K3/1
  Integrator/1 -> Add/2
  Kp1/1 -> Add/1
  Ki1/1 -> Embedded MATLAB Function1/1(din)
  K/1 -> Ki1/1, Kp1/1
  Add/1 -> K1/1
  Embedded MATLAB Function1/1(dout) -> Integrator/1
  K3/1 -> Relational Operator1/2
  Relational Operator1/1 -> Logical Operator/2
  Relational Operator/1 -> Logical Operator/1
  Logical Operator/1 -> Embedded MATLAB Function1/2(enable), D2/1
  K1/1 -> Out/1, Relational Operator/1, Relational Operator1/1

== system PhaseII_opalrt_NoProtection/SS_LocalControl/BESS2/PI_Vd6 ==
  Error : Inport
  Add : Sum
  Constant25 : Constant  Value=0.15
  D2 : Scope  NumInputPorts=2
  Embedded MATLAB Function1 : MATLAB Function  TreatAsAtomicUnit=on
  Integrator : Integrator  ZeroCross=off
  K : Gain
  K1 : Gain
  K2 : Gain  Gain=Vabc_B
  K3 : Gain  Gain=-1
  Ki1 : Gain  Gain=Ki_v
  Kp1 : Gain  Gain=Kp_v
  Logical Operator : Logic  AllPortsSameDT=off  OutDataTypeStr=boolean
  PLL : powerlib_meascontrol/PLL/PLL  Fmin=58  Par_Init=[0, 60]  ParK=[180, 3200, 1]  TcD=1e-4  MaxRateChangeFreq=12  FilterCutOffFreq=25  Ts=0  AGC=on
  Relational Operator : RelationalOperator  Operator=<  OutDataTypeStr=boolean  ZeroCross=off  RndMeth=Nearest
  Relational Operator1 : RelationalOperator  Operator=>  OutDataTypeStr=boolean  ZeroCross=off  RndMeth=Nearest
  Out : Outport
  wires:
  Error/1 -> K/1, D2/2
  Constant25/1 -> Relational Operator/2, K3/1
  Integrator/1 -> Add/2
  Kp1/1 -> Add/1
  Ki1/1 -> Embedded MATLAB Function1/1(din)
  K/1 -> Ki1/1, Kp1/1
  Add/1 -> K1/1
  Embedded MATLAB Function1/1(dout) -> Integrator/1
  K3/1 -> Relational Operator1/2
  Relational Operator1/1 -> Logical Operator/2
  Relational Operator/1 -> Logical Operator/1
  Logical Operator/1 -> Embedded MATLAB Function1/2(enable), D2/1
  K1/1 -> Out/1, Relational Operator/1, Relational Operator1/1

== system PhaseII_opalrt_NoProtection/SS_LocalControl/BESS2/PI_Vd7 ==
  Error : Inport
  T_islanding : Inport  Port=2
  Add : Sum
  Add1 : Sum  Inputs=+-
  Constant25 : Constant
  D2 : Scope  NumInputPorts=2
  Delay : Delay  DelayLength=1
  Embedded MATLAB Function1 : MATLAB Function  TreatAsAtomicUnit=on
  Integrator : Integrator  ExternalReset=falling  InitialConditionSource=external  LimitOutput=on  UpperSaturationLimit=Iabc_B*BESS_limit  LowerSaturationLimit=-Iabc_B*BESS_limit
  K : Gain
  K1 : Gain
  K2 : Gain  Gain=Vabc_B
  K3 : Gain  Gain=-1
  Ki1 : Gain  Gain=Kif
  Kp1 : Gain  Gain=Kpf
  Logical Operator : Logic  AllPortsSameDT=off  OutDataTypeStr=boolean
  PLL : powerlib_meascontrol/PLL/PLL  Fmin=58  Par_Init=[0, 60]  ParK=[180, 3200, 1]  TcD=1e-4  MaxRateChangeFreq=12  FilterCutOffFreq=25  Ts=0  AGC=on
  Relational Operator : RelationalOperator  Operator=<  OutDataTypeStr=boolean  ZeroCross=off  RndMeth=Nearest
  Relational Operator1 : RelationalOperator  Operator=>  OutDataTypeStr=boolean  ZeroCross=off  RndMeth=Nearest
  Out : Outport
  wires:
  K1/1 -> Relational Operator1/1, Relational Operator/1, Out/1
  Logical Operator/1 -> D2/1, Embedded MATLAB Function1/2(enable)
  Relational Operator/1 -> Logical Operator/1
  Relational Operator1/1 -> Logical Operator/2
  K3/1 -> Relational Operator1/2
  Embedded MATLAB Function1/1(dout) -> Integrator/1
  Add/1 -> K1/1
  K/1 -> Kp1/1, Ki1/1
  Ki1/1 -> Embedded MATLAB Function1/1(din)
  Kp1/1 -> Add1/2, Add/1
  Integrator/1 -> Add/2
  Constant25/1 -> K3/1, Relational Operator/2
  Error/1 -> D2/2, K/1
  Delay/1 -> Integrator/3
  [Ddi1] -> Add1/1
  Add1/1 -> Delay/1
  T_islanding/1 -> Integrator/2

== system PhaseII_opalrt_NoProtection/SS_LocalControl/BESS2/PI_Vd8 ==
  Error : Inport
  T_islanding : Inport  Port=2
  Add : Sum
  Add1 : Sum  Inputs=+-
  Constant25 : Constant
  D2 : Scope  NumInputPorts=2
  Delay : Delay  DelayLength=1
  Embedded MATLAB Function1 : MATLAB Function  TreatAsAtomicUnit=on
  Integrator1 : Integrator  ExternalReset=rising  InitialConditionSource=external  LimitOutput=on  UpperSaturationLimit=1  LowerSaturationLimit=-1
  K : Gain
  K1 : Gain
  K2 : Gain  Gain=Vabc_B
  K3 : Gain  Gain=-1
  Ki1 : Gain  Gain=Ki_v
  Kp1 : Gain  Gain=Kp_v
  Logical Operator : Logic  AllPortsSameDT=off  OutDataTypeStr=boolean
  PLL : powerlib_meascontrol/PLL/PLL  Fmin=58  Par_Init=[0, 60]  ParK=[180, 3200, 1]  TcD=1e-4  MaxRateChangeFreq=12  FilterCutOffFreq=25  Ts=0  AGC=on
  Relational Operator : RelationalOperator  Operator=<  OutDataTypeStr=boolean  ZeroCross=off  RndMeth=Nearest
  Relational Operator1 : RelationalOperator  Operator=>  OutDataTypeStr=boolean  ZeroCross=off  RndMeth=Nearest
  Out : Outport
  wires:
  Error/1 -> K/1, D2/2
  Constant25/1 -> Relational Operator/2, K3/1
  Integrator1/1 -> D2/1, Add/2
  Kp1/1 -> Add1/2, Add/1
  Ki1/1 -> Embedded MATLAB Function1/1(din)
  K/1 -> Ki1/1, Kp1/1
  Add/1 -> K1/1
  K3/1 -> Relational Operator1/2
  Relational Operator1/1 -> Logical Operator/2
  Relational Operator/1 -> Logical Operator/1
  Logical Operator/1 -> Embedded MATLAB Function1/2(enable)
  K1/1 -> Out/1, Relational Operator/1, Relational Operator1/1
  Embedded MATLAB Function1/1(dout) -> Integrator1/1
  [Iq_ref_ini1] -> Add1/1
  Add1/1 -> Delay/1
  Delay/1 -> Integrator1/3
  T_islanding/1 -> Integrator1/2

== system PhaseII_opalrt_NoProtection/SS_LocalControl/BESS2/PI_Vd9 ==
  Error : Inport
  T_islanding : Inport  Port=2
  Add : Sum
  Add1 : Sum  Inputs=+-
  Constant25 : Constant
  D2 : Scope  NumInputPorts=2
  Delay : Delay  DelayLength=1
  Embedded MATLAB Function1 : MATLAB Function  TreatAsAtomicUnit=on
  Integrator : Integrator  ExternalReset=falling  InitialConditionSource=external  LimitOutput=on  UpperSaturationLimit=Iabc_B*BESS_limit  LowerSaturationLimit=-Iabc_B*BESS_limit
  K : Gain
  K1 : Gain
  K2 : Gain  Gain=Vabc_B
  K3 : Gain  Gain=-1
  Ki1 : Gain  Gain=Kif
  Kp1 : Gain  Gain=Kpf
  Logical Operator : Logic  AllPortsSameDT=off  OutDataTypeStr=boolean
  PLL : powerlib_meascontrol/PLL/PLL  Fmin=58  Par_Init=[0, 60]  ParK=[180, 3200, 1]  TcD=1e-4  MaxRateChangeFreq=12  FilterCutOffFreq=25  Ts=0  AGC=on
  Relational Operator : RelationalOperator  Operator=<  OutDataTypeStr=boolean  ZeroCross=off  RndMeth=Nearest
  Relational Operator1 : RelationalOperator  Operator=>  OutDataTypeStr=boolean  ZeroCross=off  RndMeth=Nearest
  Out : Outport
  wires:
  K1/1 -> Relational Operator1/1, Relational Operator/1, Out/1
  Logical Operator/1 -> D2/1, Embedded MATLAB Function1/2(enable)
  Relational Operator/1 -> Logical Operator/1
  Relational Operator1/1 -> Logical Operator/2
  K3/1 -> Relational Operator1/2
  Embedded MATLAB Function1/1(dout) -> Integrator/1
  Add/1 -> K1/1
  K/1 -> Kp1/1, Ki1/1
  Ki1/1 -> Embedded MATLAB Function1/1(din)
  Kp1/1 -> Add1/2, Add/1
  Integrator/1 -> Add/2
  Constant25/1 -> K3/1, Relational Operator/2
  Error/1 -> D2/2, K/1
  Delay/1 -> Integrator/3
  [Dqi1] -> Add1/1
  Add1/1 -> Delay/1
  T_islanding/1 -> Integrator/2

== system PhaseII_opalrt_NoProtection/SS_LocalControl/BESS2/SW Command ==
  f : Inport
  Vd : Inport  Port=2
  SW_Ctr : Inport  Port=3
  Abs2 : Abs
  Abs3 : Abs
  Add3 : Sum  Inputs=+-
  Add4 : Sum  Inputs=+-
  Constant1 : Constant  Value=5
  Constant2 : Constant
  Constant20 : Constant  Value=0.15
  Constant21 : Constant  Value=.2
  Constant22 : Constant
  Constant23 : Constant  Value=60
  Conv : DataTypeConversion  OutDataTypeStr=double
  Counter : dspswit3/Counter  Direction=Up  CountEvent=Non-zero sample  CounterSize=User defined  MaxCount=255  InitialCount=0  Output=Hit  HitValue=50  ResetInput=on  SamplesPerFrame=1  Ts=1  CntDtype=double  HitDtype=Logical
  Counter1 : dspswit3/Counter  Direction=Up  CountEvent=Rising edge  CounterSize=User defined  MaxCount=255  InitialCount=0  Output=Count  HitValue=50  ResetInput=on  SamplesPerFrame=1  Ts=1  CntDtype=double  HitDtype=Logical
  D Latch2 : simulink_extras/Flip Flops/D Latch
  D1 : Scope  NumInputPorts=3
  D8 : Scope  NumInputPorts=3
  Delay : Delay  DelayLength=1
  Logical Operator : Logic  AllPortsSameDT=off  OutDataTypeStr=boolean
  Logical Operator{1..3,5} (4 alike) : Logic  Operator=NOT  AllPortsSameDT=off  OutDataTypeStr=boolean
  Logical Operator4 : Logic  Operator=OR  AllPortsSameDT=off  OutDataTypeStr=boolean
  Memory : Memory
  Relational Operator1 : RelationalOperator  OutDataTypeStr=boolean  RndMeth=Nearest
  Relational Operator2 : RelationalOperator  OutDataTypeStr=boolean  RndMeth=Nearest
  Relational Operator3 : RelationalOperator  OutDataTypeStr=boolean  RndMeth=Nearest
  SW_Cmd : Outport
  wires:
  Abs2/1 -> Relational Operator2/1
  Add3/1 -> Abs2/1
  Constant23/1 -> Add3/2
  Constant21/1 -> Relational Operator2/2
  Relational Operator2/1 -> D1/1, Logical Operator4/1
  Add4/1 -> Abs3/1
  Constant22/1 -> Add4/2
  D Latch2/1 -> D8/3, Logical Operator2/1
  Relational Operator3/1 -> D1/2, Logical Operator4/2
  Abs3/1 -> Relational Operator3/1
  Constant20/1 -> Relational Operator3/2
  Constant1/1 -> Relational Operator1/2
  Counter/1 -> Counter1/1
  Counter1/1 -> D1/3, Relational Operator1/1
  Logical Operator1/1 -> Counter/2
  Logical Operator4/1 -> Logical Operator5/1, Logical Operator1/1, Counter/1
  f/1 -> Add3/1
  Conv/1 -> Memory/1
  SW_Ctr/1 -> Delay/1
  Logical Operator/1 -> Conv/1
  Memory/1 -> Logical Operator3/1, D8/1
  Logical Operator2/1 -> Logical Operator/1
  Relational Operator1/1 -> D Latch2/1
  Delay/1 -> D8/2, Logical Operator/2
  Logical Operator5/1 -> Counter1/2
  Constant2/1 -> D Latch2/2
  Vd/1 -> Add4/1
  Logical Operator3/1 -> SW_Cmd/1

== system PhaseII_opalrt_NoProtection/SS_LocalControl/BESS2/Sequence decomposition1 ==
  abc : Inport
  Phase : Inport  Port=2
  Add : Sum  Inputs=+++
  Add1 : Sum
  Add2 : Sum  Inputs=+-
  Add3 : Sum
  Add4 : Sum  Inputs=-+
  Alpha-Beta-Zero to dq0 : powerlib_meascontrol/Transformations/Alpha-Beta-Zero to dq0  Alignment=90 degrees behind phase A axis
  Alpha-Beta-Zero to dq1 : powerlib_meascontrol/Transformations/Alpha-Beta-Zero to dq0  Alignment=90 degrees behind phase A axis
  Delay : Delay  DelayLength=42  InitialCondition=0
  Delay1 : Delay  DelayLength=42  InitialCondition=0
  Demux1 : Demux  Outputs=2
  Demux4 : Demux  Outputs=3
  Fcn3 : Fcn  Expr=sqrt(2/3)*(u[1]-u[2]*1/2-u[3]*1/2)
  Fcn5 : Fcn  Expr=sqrt(2/3)*(u[2]*sqrt(3)/2-u[3]*sqrt(3)/2)
  Gain1 : Gain  Gain=-1
  Gain2 : Gain  Gain=1/3
  Gain3 : Gain
  Gain{6..9} (4 alike) : Gain  Gain=1/2
  Mux : Mux  Inputs=3
  Mux1 : Mux  Inputs=3
  Mux2 : Mux  Inputs=2
  Mux3 : Mux  Inputs=3
  Pos_dq : Outport
  Neg_dq : Outport  Port=2
  zero : Outport  Port=3
  wires:
  Fcn5/1 -> Mux2/2
  Fcn3/1 -> Mux2/1
  Mux1/1 -> Fcn5/1, Fcn3/1
  Gain3/1 -> Mux/3, Mux3/3
  Phase/1 -> Alpha-Beta-Zero to dq0/2, Gain1/1
  Gain2/1 -> zero/1
  Add/1 -> Gain3/1, Gain2/1
  Gain7/1 -> Mux3/2
  Gain6/1 -> Mux3/1
  Mux3/1 -> Alpha-Beta-Zero to dq0/1
  Gain9/1 -> Mux/2
  Gain8/1 -> Mux/1
  Add3/1 -> Gain8/1
  Add4/1 -> Gain9/1
  Add2/1 -> Gain6/1
  Add1/1 -> Gain7/1
  Delay/1 -> Add1/2, Add4/1
  Delay1/1 -> Add3/2, Add2/2
  Demux4/3 -> Add/2, Mux1/3
  Demux4/2 -> Add/3, Mux1/2
  Demux4/1 -> Add/1, Mux1/1
  abc/1 -> Demux4/1
  Alpha-Beta-Zero to dq1/1 -> Neg_dq/1
  Alpha-Beta-Zero to dq0/1 -> Pos_dq/1
  Gain1/1 -> Alpha-Beta-Zero to dq1/2
  Mux/1 -> Alpha-Beta-Zero to dq1/1
  Demux1/2 -> Add1/1, Add4/2, Delay1/1
  Mux2/1 -> Demux1/1
  Demux1/1 -> Delay/1, Add3/1, Add2/1
